simulink model "Linear_PID_MODEL"  (Simulink 7.6)
settings: Solver=ode45  StartTime=0.0  StopTime=20  RelTol=1e-3
libraries: ADRC x1
settings Model: Creator=Administrator  LastModifiedBy=Administrator
settings DebuggingCC: SolverPrmCheckMsg=none

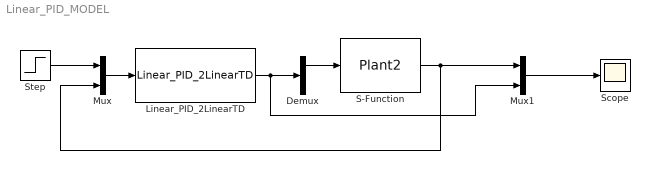
== system Linear_PID_MODEL ==
  Demux : Demux  Outputs=2
  Linear_PID_2LinearTD : ADRC/LinearPID/Linear_PID_2LinearTD  r0=2  r1=100  h=0.01  Bet=[30,50,20]
  Mux : Mux  Inputs=2
  Mux1 : Mux  Inputs=2
  S-Function : S-Function  FunctionName=Plant2  EnableBusSupport=off
  Scope : Scope
      settings: YMin=-4  YMax=3
  Step : Step  Time=0  SampleTime=0
  wires:
  Step/1 -> Mux/1
  Mux/1 -> Linear_PID_2LinearTD/1
  Mux1/1 -> Scope/1
  Linear_PID_2LinearTD/1 -> Demux/1, Mux1/2
  Demux/1 -> S-Function/1
  S-Function/1 -> Mux1/1, Mux/2
